simulink model "straightline_initial"  (R2020b)
settings: Solver=VariableStepAuto  StartTime=0.0  StopTime=inf  RelTol=1e-3
values from neighbouring files (symbols this model uses):
  z_initial = [theta0;x0;y0]    [Run_model.m]
undefined symbols (not defined in the file or in its folder): Angular, Linear
libraries: robotlib x8
settings Model: Creator=sridhar  LastModifiedBy=sridhar

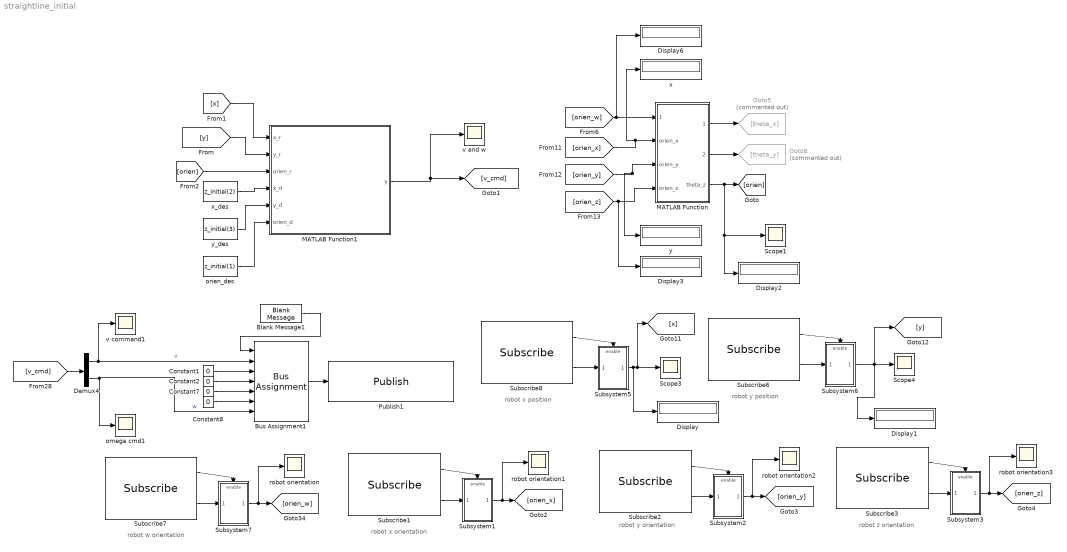
== system straightline_initial ==
  note: robot w orientation
  note: robot x orientation
  note: robot y orientation
  note: robot z orientation
  note: robot y position
  note: robot x position
   robot orientation{,1..3} (4 alike) : Scope
  Blank Message1 : robotlib/Blank Message  messageClass=Message  entityType=geometry_msgs/Twist  messageType=geometry_msgs/Twist  SampleTime=-1  legacyBusStruct=off
  Bus Assignment1 : BusAssignment  AssignedSignals=Linear.X,Linear.Y,Linear.Z,Angular.X,Angular.Y,Angular.Z
  Constant{1..2,7..8} (4 alike) : Constant  Value=0
  Demux4 : Demux  Outputs=2
  Display{,1..3,6} (5 alike) : Display
  Goto5 : Goto  Commented=on  GotoTag=theta_x
  Goto8 : Goto  Commented=on  GotoTag=theta_y
  MATLAB Function : MATLAB Function  TreatAsAtomicUnit=on
  MATLAB Function1 : MATLAB Function  TreatAsAtomicUnit=on
  Publish1 : robotlib/Publish  topicSource=Specify your own  topic=/mobile_base/commands/velocity  messageType=geometry_msgs/Twist  legacyBusStruct=off  messageQueueLength=1
  Scope1 : Scope
  Scope3 : Scope
  Scope4 : Scope
  Subscribe{1..3,6..8} (6 alike) : robotlib/Subscribe  Priority=15  topicSource=Specify your own  topic=/odom  messageType=nav_msgs/Odometry  SampleTime=-1  legacyBusStruct=off  messageQueueLength=1
  Subsystem1 : Subsystem  Priority=16
  Subsystem2 : Subsystem  Priority=16
  Subsystem3 : Subsystem  Priority=16
  Subsystem5 : Subsystem  Priority=16
  Subsystem6 : Subsystem  Priority=16
  Subsystem7 : Subsystem  Priority=16
  omega cmd1 : Scope
  orien_des : Constant  Value=z_initial(1)
  "v and w " : Scope
  v command1 : Scope
  x : Display
  x_des : Constant  Value=z_initial(2)
  y : Display
  y_des : Constant  Value=z_initial(3)
  wires:
  x_des/1 -> MATLAB Function1/4(x_d)
  [x] -> MATLAB Function1/1(x_r)
  Demux4/2 -> Bus Assignment1/7, omega cmd1/1  "w"
  Demux4/1 -> v command1/1, Bus Assignment1/2  "v"
  Blank Message1/1 -> Bus Assignment1/1
  Constant1/1 -> Bus Assignment1/3
  Constant2/1 -> Bus Assignment1/4
  Constant7/1 -> Bus Assignment1/5
  Constant8/1 -> Bus Assignment1/6
  Bus Assignment1/1 -> Publish1/1
  [v_cmd] -> Demux4/1
  Subsystem7/1(<w>) -> " robot orientation"/1, [orien_w]
  Subscribe7/2 -> Subsystem7/1(In1)
  Subscribe7/1 -> Subsystem7/Enable
  Subscribe1/1 -> Subsystem1/Enable
  Subscribe1/2 -> Subsystem1/1(In1)
  Subsystem1/1(<x>) -> [orien_x], " robot orientation1"/1
  Subsystem2/1(<y>) -> " robot orientation2"/1, [orien_y]
  Subscribe2/2 -> Subsystem2/1(In1)
  Subscribe2/1 -> Subsystem2/Enable
  Subscribe3/1 -> Subsystem3/Enable
  Subscribe3/2 -> Subsystem3/1(In1)
  Subsystem3/1(<Z>) -> [orien_z], " robot orientation3"/1
  Subscribe6/1 -> Subsystem6/Enable
  Subscribe8/1 -> Subsystem5/Enable
  Subscribe8/2 -> Subsystem5/1(In1)
  Subsystem5/1(<X>) -> Scope3/1, [x], Display/1
  Subsystem6/1(<Y>) -> Scope4/1, Display1/1, [y]
  Subscribe6/2 -> Subsystem6/1(In1)
  [orien_w] -> Display6/1, MATLAB Function/1(orien_w)
  [orien_x] -> MATLAB Function/2(orien_x), x/1
  [orien_y] -> MATLAB Function/3(orien_y), y/1
  [orien_z] -> MATLAB Function/4(orien_z), Display3/1
  MATLAB Function/1(theta_x) -> Goto5/1
  MATLAB Function/2(theta_y) -> Goto8/1
  MATLAB Function/3(theta_z) -> [orien], Scope1/1, Display2/1
  MATLAB Function1/1(y) -> "v and w "/1, [v_cmd]
  [y] -> MATLAB Function1/2(y_r)
  [orien] -> MATLAB Function1/3(orien_r)
  orien_des/1 -> MATLAB Function1/6(orien_d)
  y_des/1 -> MATLAB Function1/5(y_d)

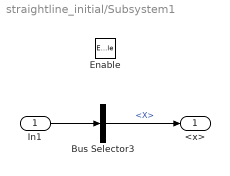
== system straightline_initial/Subsystem1 ==
  In1 : Inport
  Enable : EnablePort
  Bus Selector3 : BusSelector  OutputSignals=Pose.Pose.Orientation.X
  <x> : Outport
  wires:
  Bus Selector3/1 -> <x>/1  "<X>"
  In1/1 -> Bus Selector3/1

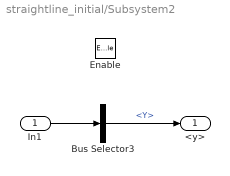
== system straightline_initial/Subsystem2 ==
  In1 : Inport
  Enable : EnablePort
  Bus Selector3 : BusSelector  OutputSignals=Pose.Pose.Orientation.Y
  <y> : Outport
  wires:
  In1/1 -> Bus Selector3/1
  Bus Selector3/1 -> <y>/1  "<Y>"

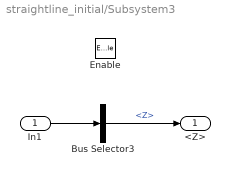
== system straightline_initial/Subsystem3 ==
  In1 : Inport
  Enable : EnablePort
  Bus Selector3 : BusSelector  OutputSignals=Pose.Pose.Orientation.Z
  <Z> : Outport
  wires:
  Bus Selector3/1 -> <Z>/1  "<Z>"
  In1/1 -> Bus Selector3/1

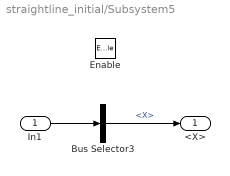
== system straightline_initial/Subsystem5 ==
  In1 : Inport
  Enable : EnablePort
  Bus Selector3 : BusSelector  OutputSignals=Pose.Pose.Position.X
  <X> : Outport
  wires:
  In1/1 -> Bus Selector3/1
  Bus Selector3/1 -> <X>/1  "<X>"

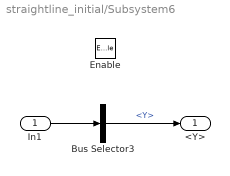
== system straightline_initial/Subsystem6 ==
  In1 : Inport
  Enable : EnablePort
  Bus Selector3 : BusSelector  OutputSignals=Pose.Pose.Position.Y
  <Y> : Outport
  wires:
  In1/1 -> Bus Selector3/1
  Bus Selector3/1 -> <Y>/1  "<Y>"

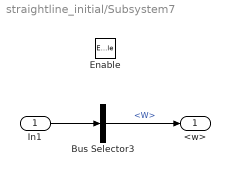
== system straightline_initial/Subsystem7 ==
  In1 : Inport
  Enable : EnablePort
  Bus Selector3 : BusSelector  OutputSignals=Pose.Pose.Orientation.W
  <w> : Outport
  wires:
  In1/1 -> Bus Selector3/1
  Bus Selector3/1 -> <w>/1  "<W>"

== matlab function straightline_initial/MATLAB Function ==
  data: orien_w input; orien_x input; theta_x output; theta_y output; orien_y input; orien_z input; theta_z output
function [theta_x, theta_y, theta_z] = fcn(orien_w, orien_x, orien_y, orien_z)
% input is [w x y z] 
% output is [z y x]

quat = [orien_w, orien_x, orien_y, orien_z];
eul = quat2eul(quat);

theta_x = eul(3);
theta_y = eul(2);
theta_z = eul(1);

== matlab function straightline_initial/MATLAB Function1 ==
  data: x_r input; y_r input; orien_r input; x_d input; y_d input; y output; orien_d input
function y = fcn(x_r, y_r, orien_r, x_d, y_d, orien_d)

orien_diff = abs(orien_d-orien_r);
if (orien_diff > 0.003)
    w=0.1;
    v=0.0;
% elseif (orien_r<orien_d)
%     w = 0.01;
%     v = 0;
% elseif (orien_r>orien_d)
%     w = -0.01;
%     v = 0; 
else
    w = 0;
    v = 0;
end

% x_diff = abs(x_d-x_r);
% if (orien_r < 0.1) && (x_diff>0.1*abs(r))
%     w = 0.0;
%     v = 0.1;
% elseif (x_diff <= 0.15*abs(r)) && (orien_r <= 1.5)
%     w= 0.2;
%     v= 0;
% else 
%     w = 0.001;
%     v = 0.001;
% end

y = [v; w];
